simulink model "hybrid"  (R2021b)
settings: Solver=ode3  StartTime=0.0  StopTime=100  FixedStep=0.001  RelTol=1e-3
undefined symbols (not defined in the file or in its folder): HIL, K
libraries: quarc_library x4
settings Model: ExtModeTrigDuration=100000  Creator=h.kaitang  LastModifiedBy=hukai
settings SolverCC: AlgebraicLoopSolver=TrustRegion  PositivePriorityOrder=on
settings DebuggingCC: SFMachineParentedDataDiag=warning  ArithmeticOperatorsInVariantConditions=warning
settings SFSimCC: SimUseLocalCustomCode=off  CustomCodeUndefinedFunction=UseInterfaceOnly
settings RTWCC: Description=QUARC Win64 Target Using Toolchain  SystemTargetFile=quarc_win64.tlc  TemplateMakefile=quarc_default_tmf  RTWUseLocalCustomCode=off  Toolchain=QUARC win64 | nmake (64-bit Windows)  BuildConfiguration=Faster Runs
settings CodeAppCC: StateflowObjectComments=on
settings STFCustomTargetCC: TargetLangStandard=C99 (ISO)  ConcurrentExecutionCompliant=on  UseToolchainInfoCompliant=on  SystemTargetFile=quarc_win64.tlc
settings GRTTargetCC: ParMdlRefBuildCompliant=off  CompOptLevelCompliant=off  CombineOutputUpdateFcns=off  MatFileLogging=off  CPPClassGenCompliant=off  GRTInterface=on  ExtMode=on  ExtModeMexFile=quarc_comm
settings ConfigComp: CovMetricSettings=dswe

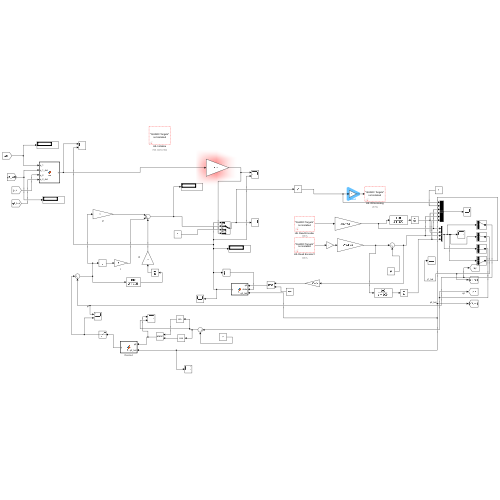
[thumbnail: Simulink's stored preview of the top-level diagram]
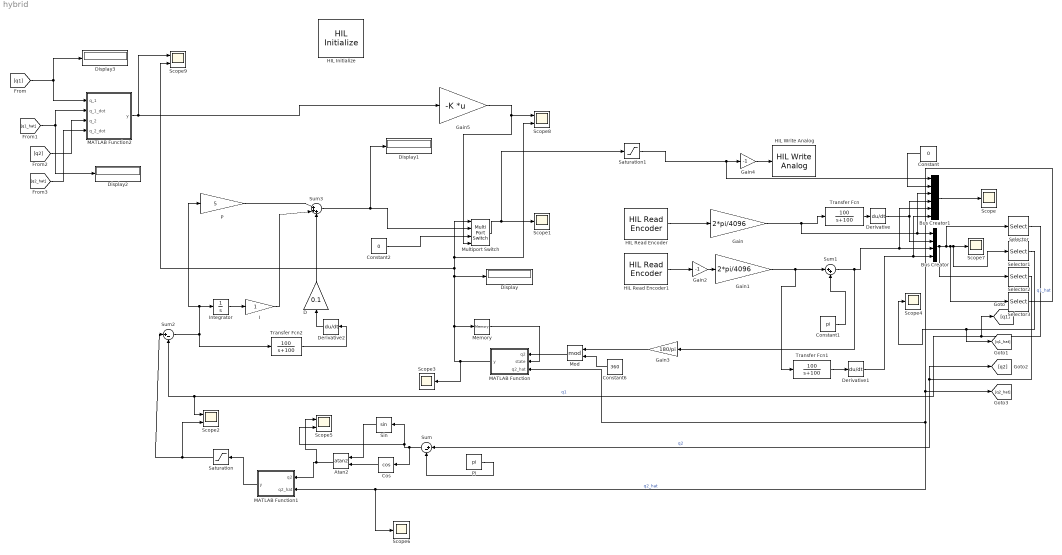
== system hybrid ==
  Atan2 : Trigonometry  Operator=atan2
  Bus Creator : BusCreator  Inputs=4
  Bus Creator1 : BusCreator  Inputs=6
  Constant : Constant  Value=0
  Constant1 : Constant  Value=pi
  Constant2 : Constant  Value=0
  Constant6 : Constant  Value=360
  Cos : Trigonometry  Operator=cos
  D : Gain  Gain=0.1
  Derivative : Derivative
  Derivative1 : Derivative
  Derivative2 : Derivative
  Display{,1..3} (4 alike) : Display
  Gain : Gain  Gain=2*pi/4096
  Gain1 : Gain  Gain=2*pi/4096
  Gain2 : Gain  Gain=-1
  Gain3 : Gain  Gain=180/pi
  Gain4 : Gain  Gain=-1
  Gain5 : Gain  Gain=-K  Multiplication=Matrix(K*u)
  HIL Initialize : quarc_library/Data Acquisition/Generic/Configuration/HIL Initialize  object_name=HIL-1  board_type=q2_usb  board_number=0  board_options=d0=digital;d1=digital;led=auto;update_rate=normal;decimation=1  exclusive=off  active=on  hardware_clocks=[0]  clock_modes=[]  initial_clock_frequencies=[]  set_clock_params_at_start=off  set_clock_params_at_switch_in=off  set_clock_frequencies_at_start=off  set_clock_frequencies_at_switch_in=off  analog_input_channels=[0:1]  analog_input_configurations=[]  analog_input_maximums=10  analog_input_minimums=-10  set_analog_input_params_at_start=on  set_analog_input_params_at_switch_in=off  analog_output_channels=[0:1]  analog_output_maximums=10  analog_output_minimums=-10  initial_analog_outputs=[0]  final_analog_outputs=[0]  watchdog_analog_outputs=0  set_analog_output_params_at_start=on  set_analog_output_params_at_switch_in=off  set_analog_outputs_at_start=on  set_analog_outputs_at_switch_in=off  set_analog_outputs_at_terminate=on  set_analog_outputs_at_switch_out=off  set_analog_outputs_on_watchdog=off  digital_input_channels=[]  digital_output_channels=[]  digital_output_configuration=[]  initial_digital_outputs=[1]  final_digital_outputs=[1]  watchdog_digital_outputs=[1]  set_digital_output_params_at_start=off  set_digital_output_params_at_switch_in=off  set_digital_outputs_at_start=on  set_digital_outputs_at_switch_in=off  set_digital_outputs_at_terminate=on  set_digital_outputs_at_switch_out=off  set_digital_outputs_on_watchdog=off  encoder_channels=[0:1]  quadrature=[4]  encoder_filter_frequency=[]  initial_encoder_counts=[0]  set_encoder_params_at_start=on  set_encoder_params_at_switch_in=off  set_encoder_counts_at_start=on  set_encoder_counts_at_switch_in=off  pwm_channels=[]  pwm_modes=[0]  pwm_frequency=1/0.020  pwm_configuration=[]  pwm_alignment=[]  pwm_polarity=[]  pwm_leading_deadband=[]  pwm_trailing_deadband=[]  initial_pwm_outputs=[0]  final_pwm_outputs=[0]  watchdog_pwm_outputs=[0]  set_pwm_params_at_start=on  set_pwm_params_at_switch_in=off  set_pwm_outputs_at_start=on  set_pwm_outputs_at_switch_in=off  set_pwm_outputs_at_terminate=on  set_pwm_outputs_at_switch_out=off  set_pwm_outputs_on_watchdog=off  other_output_channels=[]  initial_other_outputs=[]  final_other_outputs=[]  watchdog_other_outputs=[]  set_other_outputs_at_start=off  set_other_outputs_at_switch_in=off  set_other_outputs_at_terminate=off  set_other_outputs_at_switch_out=off  set_other_outputs_on_watchdog=off
  HIL Read Encoder : quarc_library/Data Acquisition/Generic/Immediate I//O/HIL Read Encoder  object_name=HIL-1  channels=0  sample_time=qc_get_step_size  active=on  vector_output=off  data_type_mode=Inherit via back propagation  data_type=double
  HIL Read Encoder1 : quarc_library/Data Acquisition/Generic/Immediate I//O/HIL Read Encoder  object_name=HIL-1  channels=1  sample_time=qc_get_step_size  active=on  vector_output=off  data_type_mode=Inherit via back propagation  data_type=double
  HIL Write Analog : quarc_library/Data Acquisition/Generic/Immediate I//O/HIL Write Analog  object_name=HIL-1  channels=0  sample_time=-1  active=off  vector_input=off
  I : Gain
  Integrator : Integrator
  MATLAB Function : MATLAB Function  TreatAsAtomicUnit=on
  MATLAB Function1 : MATLAB Function  Tag=Desired  TreatAsAtomicUnit=on
      settings: AttributesFormatString=%<Tag>
  MATLAB Function2 : MATLAB Function  TreatAsAtomicUnit=on
  Memory : Memory  InitialCondition=1
  Mod : Math  Operator=mod  SaturateOnIntegerOverflow=on
  Multiport Switch : MultiPortSwitch
  P : Gain  Gain=5
  Pi : Constant  Value=pi  OutDataTypeStr=Inherit: Inherit via back propagation
  Saturation : Saturate  UpperLimit=0.8  LowerLimit=-0.8
  Saturation1 : Saturate  UpperLimit=10  LowerLimit=-10
  Scope{,1,3..4,6..7} (6 alike) : Scope
  Scope{2,5,8..9} (4 alike) : Scope  NumInputPorts=2
  Selector : Selector  InputPortWidth=4  IndexOptions=Index vector (dialog)  Indices=1  OutputSizes=1
  Selector1 : Selector  InputPortWidth=4  IndexOptions=Index vector (dialog)  Indices=2  OutputSizes=1
  Selector2 : Selector  InputPortWidth=4  IndexOptions=Index vector (dialog)  Indices=3  OutputSizes=1
  Selector3 : Selector  InputPortWidth=4  IndexOptions=Index vector (dialog)  Indices=4  OutputSizes=1
  Sin : Trigonometry
  Sum : Sum  Inputs=|+-
  Sum1 : Sum  Inputs=|++
  Sum2 : Sum  Inputs=|+-
  Sum3 : Sum  Inputs=|+++
  Transfer Fcn : TransferFcn  Numerator=100  Denominator=[1 100]
  Transfer Fcn1 : TransferFcn  Numerator=100  Denominator=[1 100]
  Transfer Fcn2 : TransferFcn  Numerator=100  Denominator=[1 100]
  wires:
  Bus Creator/1 -> Selector2/1, Selector/1, Selector3/1, Selector1/1, Scope7/1
  Transfer Fcn/1 -> Derivative/1
  Gain2/1 -> Gain1/1
  HIL Read Encoder1/1 -> Gain2/1
  HIL Read Encoder/1 -> Gain/1
  Constant1/1 -> Sum1/2
  Sum1/1 -> Bus Creator1/5, Bus Creator/3, Gain3/1
  Gain3/1 -> Mod/1
  Multiport Switch/1 -> Saturation1/1, Scope1/1
  MATLAB Function/1(y) -> Scope3/1, Memory/1, Scope9/2, Scope8/2, Multiport Switch/1, Display/1
  Memory/1 -> MATLAB Function/2(state)
  Constant6/1 -> Mod/2
  Mod/1 -> MATLAB Function/1(q2)
  Gain1/1 -> Transfer Fcn1/1, Sum1/1
  Gain/1 -> Bus Creator1/3, Bus Creator/1, Transfer Fcn/1
  Transfer Fcn1/1 -> Derivative1/1
  Gain4/1 -> HIL Write Analog/1
  Saturation1/1 -> Bus Creator1/1, Gain4/1
  Integrator/1 -> I/1
  Transfer Fcn2/1 -> Derivative2/1
  D/1 -> Sum3/3
  Sum2/1 -> P/1, Integrator/1, Transfer Fcn2/1
  I/1 -> Sum3/2
  P/1 -> Sum3/1
  Derivative2/1 -> D/1
  MATLAB Function1/1(y) -> Saturation/1
  Saturation/1 -> Scope2/2, Sum2/1
  Sum3/1 -> Display1/1, Multiport Switch/2
  Derivative/1 -> Bus Creator/2, Bus Creator1/4
  Selector/1 -> Sum2/2, Scope2/1, [q1]  "q1"
  Selector1/1 -> Scope4/1, [q1_hat]  "q1_hat"
  Selector3/1 -> [q2_hat], Scope6/1, MATLAB Function1/2(q2_hat), MATLAB Function/3(q2_hat)  "q2_hat"
  Sum/1 -> Scope5/2, Sin/1, Cos/1
  Atan2/1 -> Scope5/1, MATLAB Function1/1(q2)
  Sin/1 -> Atan2/1
  Cos/1 -> Atan2/2
  Selector2/1 -> [q2], Sum/1  "q2"
  Pi/1 -> Sum/2
  Bus Creator1/1 -> Scope/1
  Constant/1 -> Bus Creator1/2
  [q1_hat] -> Display2/1, MATLAB Function2/2(q_1_dot)
  [q2] -> MATLAB Function2/3(q_2)
  [q2_hat] -> MATLAB Function2/4(q_2_dot)
  MATLAB Function2/1(y) -> Scope9/1, Gain5/1
  Gain5/1 -> Multiport Switch/4, Scope8/1
  Constant2/1 -> Multiport Switch/3
  [q1] -> Display3/1, MATLAB Function2/1(q_1)
  Derivative1/1 -> Bus Creator1/6, Bus Creator/4

== matlab function hybrid/MATLAB Function1 ==
  data: q2 input; y output; q2_hat input
function y = fcn(q2,q2_hat)
k1 = 1;
k2 = 0;
y = k1*q2+k2*q2_hat;

== matlab function hybrid/MATLAB Function ==
  data: q2 input; y output; state input; q2_hat input
function y = fcn(q2,state,q2_hat)
% in state 1
if (q2 > 170) && (q2 < 190) && (state == 2) &&(abs(q2_hat)<0.5)
    y = 1;
elseif ((q2 < 20) && (q2 >0) && (state ==1)) || ((q2 >340) && (q2 <360) && (state ==1))
    y = 3;
elseif ((q2 > 20) && (state ==3))&& (q2 < 340)
    y = 2;
else 
    y =state;
end

%atan(sin(q2), cos(q2))

== matlab function hybrid/MATLAB Function2 ==
  data: y output; q_1 input; q_1_dot input; q_2 input; q_2_dot input
function y = fcn(q_1,q_1_dot,q_2,q_2_dot)
q_2 = atan2(sin(q_2),cos(q_2));
q_hat = [q_1;q_1_dot;q_2;q_2_dot];
y = q_hat;
